simulink model "GAPID_NNPID_COMP"  (R2018a)
settings: Solver=FixedStepAuto  StartTime=0.0  StopTime=100  FixedStep=1e-3  RelTol=1e-3
model workspace (MAT data in the model file):
  Af = 3
  Cd = 0.38
  Cr = 0.01
  DrCycles.C505 = [0 1 2 3 4 5 6 7 8 9 10 11 ... (1012 elements, 506x2)]
  DrCycles.FTP = [0 1 2 3 4 5 6 7 8 9 10 11 ... (4956 elements, 2478x2)]
  DrCycles.UDDS = [0 1 2 3 4 5 6 7 8 9 10 11 ... (2746 elements, 1373x2)]
  DrCycles.HWFET = [0 1 2 3 4 5 6 7 8 9 10 11 ... (1532 elements, 766x2)]
  DrCycles.US06 = [0 1 2 3 4 5 6 7 8 9 10 11 ... (1194 elements, 597x2)]
  DrCycles.US06City = [0 1 2 3 4 5 6 7 8 9 10 11 ... (466 elements, 233x2)]
  DrCycles.US06Hwy = [0 1 2 3 4 5 6 7 8 9 10 11 ... (742 elements, 371x2)]
  I = 1
  Kbr = 5000
  M = 1500
  P = 20
  Sig = Simulink.Signal
  Sig.DataType = 'auto'
  Sig.Dimensions = -1
  Sig.DimensionsMode = 'auto'
  Sig.Complexity = 'auto'
  Sig.SampleTime = -1
  Sig.SamplingMode = 'auto'
  Sig1 = Simulink.Signal
  Sig1.DataType = 'auto'
  Sig1.Dimensions = -1
  Sig1.DimensionsMode = 'auto'
  Sig1.Complexity = 'auto'
  Sig1.SampleTime = -1
  Sig1.SamplingMode = 'auto'
  TimeHWFET = 765
  TimeUDDS = 1372
  TimeUS06 = 596
  W_h_o = [-9.95144559352  0.700876377684  31237.1112906; -121.542629392  0.870455912648  31044.7209619; -122.360742678  0.0476540509418  31044.6526126; -122.423418817  0.59044997874  31044.0707224]
  W_i_h = [0.80068585569  0.0488168547579  0.252518618973  0.0925761755134; 0.988834029296  0.225213340605  0.654342062876  0.334021271958; 0.439228284919  0.581023041467  0.0600961897607  0.651090707805; -0.495532270503  0.596404398277  0.940082136994  0.486403351376]
  axle_b = 10
  axle_k = 5000
  bevAxle_wc = 400
  bevNp = 2
  bevNs = 30
  diffRatio = 3.4
  g = 9.81
  m = 1500
  motorMaxTorqueNm = [500 500 500 500 500 500 416.666666667 357.142857143 312.5 277.777777778 250 227.272727273 208.333333333 192.307692308 178.571428571 166.666666667]
  motorSpeedRadPs = [0 40 80 120 160 200 240 280 320 360 400 440 480 520 560 600]
  rho = 1.28
  theta = 45
  vehicleMass = 1500
  wheelRadius = 0.35
values from neighbouring files (symbols this model uses):
  Kd = reshape(Kd,D1,D2,D3)    [Launch_Comparison.m]
  Ki = reshape(Ki,D1,D2,D3)    [Launch_Comparison.m]
  Kp = reshape(Kp,D1,D2,D3)    [Launch_Comparison.m]
  lr = 0.8    [Launch_Comparison.m]
  Theta = data(:,4)    [Launch_Comparison.m]
  Vref = data(:,6)    [Launch_Comparison.m]
  Vwind = data(:,5)    [Launch_Comparison.m]
undefined symbols (not defined in the file or in its folder): sigbuilder_block
libraries: simulink x4, autolibdatasheetbattery x2, autolibmappedmotor x2, autolibsharedcoupling x2, autolibshareddiff x2, autolibshared x2, Wheels_Driver_VehDyn_Lib x2
settings Model: OrderedModelArguments=off  Creator=Yacine.Kebbati  LastModifiedBy=yassi
settings DataIOCC: ReturnWorkspaceOutputs=on
settings SFSimCC: SimUseLocalCustomCode=on
settings RTWCC: RTWUseLocalCustomCode=on

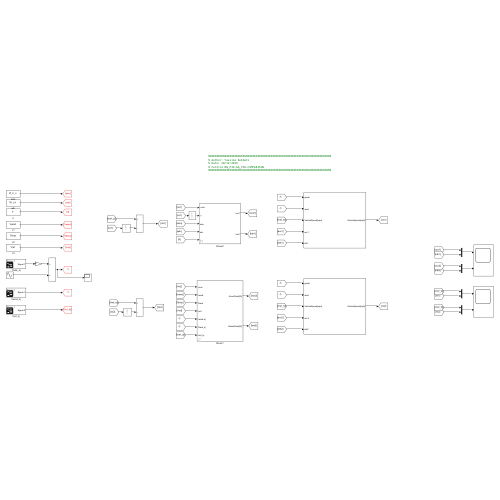
[thumbnail: Simulink's stored preview of the top-level diagram]
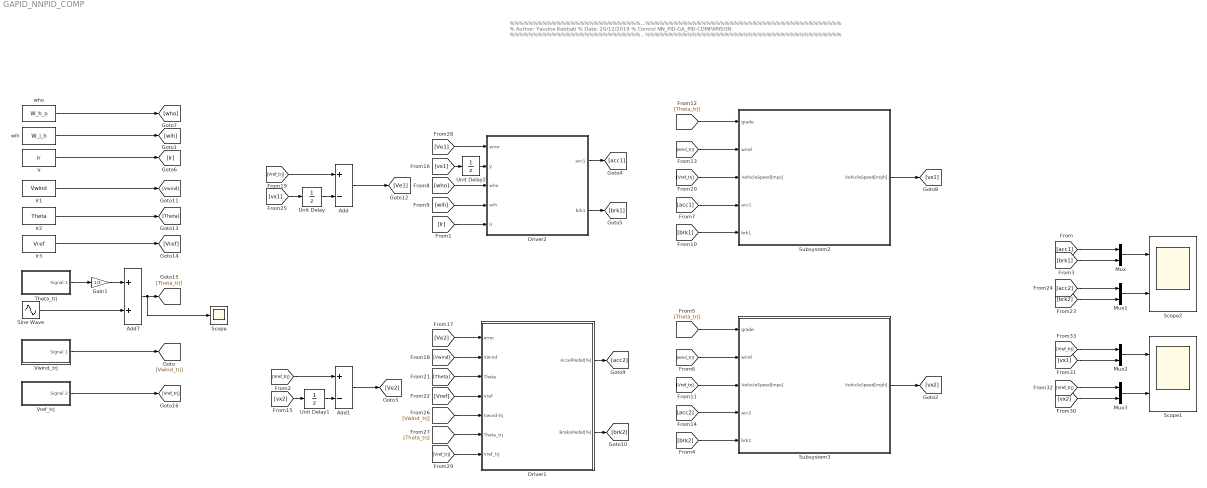
== system GAPID_NNPID_COMP ==
  note: %%%%%%%%%%%%%%%%%%%%%%%%%%%%%%%%%%%%%%%%%%%%%%%%%%%%%%%%%%%%%%%%%%%%%%%%%%%
      | % Author: Yassine Kebbati
      | % Date: 20/12/2019
      | % Control NN_PID-GA_PID-COMPARISON
      | %%%%%%%%%%%%%%%%%%%%%%%%%%%%%%%%%%%%%%%%%%%%%%%%%%%%%%%%%%%%%%%%%%%%%%%%%%%
  Add : Sum  Inputs=+-
  Add1 : Sum  Inputs=+-
  Add7 : Sum
  Driver1 : Subsystem  AncestorBlock=Wheels_Driver_VehDyn_Lib/Driver
  Driver2 : Subsystem  AncestorBlock=Wheels_Driver_VehDyn_Lib/Driver
  Gain1 : Gain  Gain=1/3
  Mux{,1..3} (4 alike) : Mux  Inputs=2
  Scope : Scope
  Scope1 : Scope  NumInputPorts=2
  Scope2 : Scope  NumInputPorts=2
  Sine Wave : Sin  Amplitude=4  Frequency=0.2  SampleTime=0
  Subsystem2 : Subsystem
  Subsystem3 : Subsystem
  Theta_trj : Subsystem  Tag=STV Subsys  LoadFcn=sigbuilder_block('load');  StartFcn=sigbuilder_block('start');  StopFcn=sigbuilder_block('stop');  ClipboardFcn=sigbuilder_block('clipboard');  mask(Sigbuilder block){tuvar=[0:10]}
      mask help: Simulink:masks:SigbuilderBlock_MD
      mask init:
      | if ~strcmp(get_param(bdroot(gcbh),'SimulationStatus'),'stopped') tuvar = sigbuilder_block('maskInit'); end
      settings: CopyFcn=sigbuilder_block('copy');  DeleteFcn=sigbuilder_block('delete');  ModelCloseFcn=sigbuilder_block('modelClose');  PreSaveFcn=sigbuilder_block('preSave');  PauseFcn=sigbuilder_block('pause');  ContinueFcn=sigbuilder_block('continue');  NameChangeFcn=sigbuilder_block('namechange');  OpenFcn=sigbuilder_block('open',[6 30 1428 681.75 ]);  CloseFcn=sigbuilder_block('close');
      mask Display: plot(0, 0, 100, 100,[2, 2, 32, 32, 2], [68, 8, 8, 68, 68],[32, 2], [38, 38], [32, 19, 2],[53, 60, 44], [32, 17, 17, 2],[16, 16, 31, 31]);txt = getActiveGroup(gcbh);text(2, 100, txt,'verticalAlignment', 'top');
  Unit Delay : UnitDelay  SampleTime=-1  HasFrameUpgradeWarning=on
  Unit Delay1 : UnitDelay  SampleTime=-1  HasFrameUpgradeWarning=on
  Unit Delay2 : UnitDelay  SampleTime=-1  HasFrameUpgradeWarning=on
  Vref_trj : Subsystem  Tag=STV Subsys  LoadFcn=sigbuilder_block('load');  StartFcn=sigbuilder_block('start');  StopFcn=sigbuilder_block('stop');  ClipboardFcn=sigbuilder_block('clipboard');  mask(Sigbuilder block){tuvar=[0:10]}
      mask help: Simulink:masks:SigbuilderBlock_MD
      mask init:
      | if ~strcmp(get_param(bdroot(gcbh),'SimulationStatus'),'stopped') tuvar = sigbuilder_block('maskInit'); end
      settings: CopyFcn=sigbuilder_block('copy');  DeleteFcn=sigbuilder_block('delete');  ModelCloseFcn=sigbuilder_block('modelClose');  PreSaveFcn=sigbuilder_block('preSave');  PauseFcn=sigbuilder_block('pause');  ContinueFcn=sigbuilder_block('continue');  NameChangeFcn=sigbuilder_block('namechange');  OpenFcn=sigbuilder_block('open',[0 36 1920 986.25 ]);  CloseFcn=sigbuilder_block('close');
      mask Display: plot(0, 0, 100, 100,[2, 2, 32, 32, 2], [68, 8, 8, 68, 68],[32, 2], [38, 38], [32, 19, 2],[53, 60, 44], [32, 17, 17, 2],[16, 16, 31, 31]);txt = getActiveGroup(gcbh);text(2, 100, txt,'verticalAlignment', 'top');
  Vwind_trj : Subsystem  Tag=STV Subsys  LoadFcn=sigbuilder_block('load');  StartFcn=sigbuilder_block('start');  StopFcn=sigbuilder_block('stop');  ClipboardFcn=sigbuilder_block('clipboard');  mask(Sigbuilder block){tuvar=[0:10]}
      mask help: Simulink:masks:SigbuilderBlock_MD
      mask init:
      | if ~strcmp(get_param(bdroot(gcbh),'SimulationStatus'),'stopped') tuvar = sigbuilder_block('maskInit'); end
      settings: CopyFcn=sigbuilder_block('copy');  DeleteFcn=sigbuilder_block('delete');  ModelCloseFcn=sigbuilder_block('modelClose');  PreSaveFcn=sigbuilder_block('preSave');  PauseFcn=sigbuilder_block('pause');  ContinueFcn=sigbuilder_block('continue');  NameChangeFcn=sigbuilder_block('namechange');  OpenFcn=sigbuilder_block('open',[140.25 245.25 1428 681.75 ]);  CloseFcn=sigbuilder_block('close');
      mask Display: plot(0, 0, 100, 100,[2, 2, 32, 32, 2], [68, 8, 8, 68, 68],[32, 2], [38, 38], [32, 19, 2],[53, 60, 44], [32, 17, 17, 2],[16, 16, 31, 31]);txt = getActiveGroup(gcbh);text(2, 100, txt,'verticalAlignment', 'top');
  lr : Constant  Value=lr  SampleTime=-1
  lr1 : Constant  Value=Vwind  SampleTime=-1
  lr2 : Constant  Value=Theta  SampleTime=-1
  lr3 : Constant  Value=Vref  SampleTime=-1
  who : Constant  Value=W_h_o  SampleTime=-1
  wih : Constant  Value=W_i_h  SampleTime=-1
  wires:
  [Theta_trj] -> Subsystem2/1(grade)
  Driver2/1(acc1) -> [acc1]
  [vx1] -> Unit Delay/1
  Add/1 -> [Ve1]
  [Vref_trj] -> Subsystem2/3(VehicleSpeed[mps])
  [Vref_trj] -> Add/1
  [acc1] -> Subsystem2/4(acc1)
  [brk1] -> Subsystem2/5(brk1)
  Subsystem2/1(VehicleSpeed[mph]) -> [vx1]
  Driver2/2(brk1) -> [brk1]
  [wind_trj] -> Subsystem2/2(wind)
  [vx1] -> Unit Delay2/1
  [Ve1] -> Driver2/1(" error")
  who/1 -> [who]
  wih/1 -> [wih]
  lr/1 -> [lr]
  [who] -> Driver2/3(who)
  [wih] -> Driver2/4(wih)
  [lr] -> Driver2/5(lr)
  Mux1/1 -> Scope2/2
  Mux/1 -> Scope2/1
  [acc1] -> Mux/1
  [brk1] -> Mux/2
  Subsystem3/1(VehicleSpeed[mph]) -> [vx2]
  [acc2] -> Subsystem3/4(acc2)
  [wind_trj] -> Subsystem3/2(wind)
  [brk2] -> Subsystem3/5(brk2)
  [Theta_trj] -> Subsystem3/1(grade)
  [Vref_trj] -> Subsystem3/3(VehicleSpeed[mps])
  [Vref_trj] -> Add1/1
  Add1/1 -> [Ve2]
  [vx2] -> Unit Delay1/1
  [Ve2] -> Driver1/1(" error")
  Driver1/1(AccelPedal[%]) -> [acc2]
  Driver1/2(BrakePedal[%]) -> [brk2]
  [Vwind] -> Driver1/2(Vwind)
  [Theta] -> Driver1/3(Theta)
  [Vref] -> Driver1/4(Vref)
  [acc2] -> Mux1/1
  [brk2] -> Mux1/2
  lr1/1 -> [Vwind]
  lr3/1 -> [Vref]
  lr2/1 -> [Theta]
  [Vwind_trj] -> Driver1/5(Vwind-trj)
  [Theta_trj] -> Driver1/6(Theta_trj)
  [Vref_trj] -> Driver1/7(Vref_trj)
  Sine Wave/1 -> Add7/2
  Gain1/1 -> Add7/1
  Theta_trj/1(Signal 1) -> Gain1/1
  Add7/1 -> Scope/1, [Theta_trj]
  Vwind_trj/1(Signal 1) -> [Vwind_trj]
  Vref_trj/1(Signal 2) -> [Vref_trj]
  Unit Delay/1 -> Add/2
  Unit Delay1/1 -> Add1/2
  Unit Delay2/1 -> Driver2/2(" y")
  [vx2] -> Mux3/2
  [Vref_trj] -> Mux3/1
  [vx1] -> Mux2/2
  [Vref_trj] -> Mux2/1
  Mux2/1 -> Scope1/1
  Mux3/1 -> Scope1/2

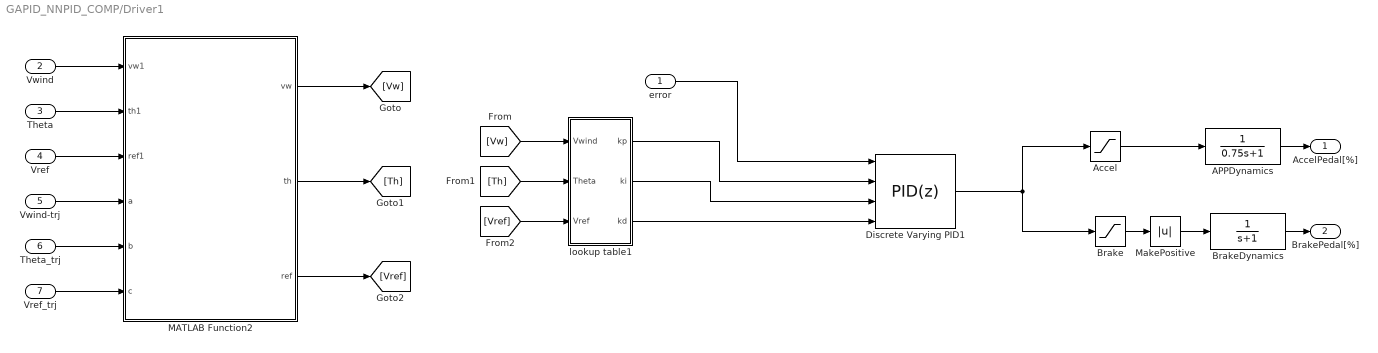
== system GAPID_NNPID_COMP/Driver1 ==
  " error" : Inport
  Vwind : Inport  Port=2
  Theta : Inport  Port=3
  Vref : Inport  Port=4
  Vwind-trj : Inport  Port=5
  Theta_trj : Inport  Port=6
  Vref_trj : Inport  Port=7
  APPDynamics : TransferFcn  Denominator=[0.75 1]
  Accel : Saturate  UpperLimit=100  LowerLimit=0
  Brake : Saturate  UpperLimit=0  LowerLimit=-100
  BrakeDynamics : TransferFcn  Denominator=[1 1]
  Discrete Varying PID1 : simulink/Continuous/PID Controller  Controller=PID  Form=Parallel  TimeDomain=Discrete-time  SampleTime=-1  IntegratorMethod=Forward Euler  ControllerParametersSource=external  P=1  I=1  D=0  N=100  UseFilter=off  TunerSelectOption=Transfer Function Based (PID Tuner App)  InitialConditionSource=internal  InitialConditionForIntegrator=0  InitialConditionForFilter=0  DifferentiatorICPrevScaledInput=0  ExternalReset=none  TrackingMode=off  Kt=1  LimitOutput=off  UpperSaturationLimit=100  LowerSaturationLimit=-100  LinearizeAsGain=on  AntiWindupMode=none  Kb=1  POutMin=[]  POutMax=[]  IOutMin=[]  IOutMax=[]  DOutMin=[]  DOutMax=[]  NOutMin=[]  NOutMax=[]  SumOutMin=[]  SumOutMax=[]  SaturationOutMin=[]  SaturationOutMax=[]  PParamMin=[]  PParamMax=[]  IParamMin=[]  IParamMax=[]  DParamMin=[]  DParamMax=[]  NParamMin=[]  NParamMax=[]  KbParamMin=[]  KbParamMax=[]  KtParamMin=[]  KtParamMax=[]  KbOutMin=[]  KbOutMax=[]  KtOutMin=[]  KtOutMax=[]  IntegratorOutMin=[]  IntegratorOutMax=[]  FilterOutMin=[]  FilterOutMax=[]  SumI1OutMin=[]  SumI1OutMax=[]  SumI2OutMin=[]  SumI2OutMax=[]  SumI3OutMin=[]  SumI3OutMax=[]  SumDOutMin=[]  SumDOutMax=[]  DifferentiatorOutMin=[]  DifferentiatorOutMax=[]  FilterDiffOutCoefMin=[]  FilterDiffOutCoefMax=[]  ReciprocalOutMin=[]  ReciprocalOutMax=[]  SumDenOutMin=[]  SumDenOutMax=[]  SumNumOutMin=[]  SumNumOutMax=[]  DivideOutMin=[]  DivideOutMax=[]  IntegratorContinuousStateAttributes=''  IntegratorStateMustResolveToSignalObject=off  IntegratorRTWStateStorageClass=Auto  FilterContinuousStateAttributes=''  FilterStateMustResolveToSignalObject=off  FilterRTWStateStorageClass=Auto
  MATLAB Function2 : MATLAB Function  TreatAsAtomicUnit=on
  MakePositive : Abs
  lookup table1 : Subsystem
  AccelPedal[%] : Outport  VectorParamsAs1DForOutWhenUnconnected=off
  BrakePedal[%] : Outport  Port=2  VectorParamsAs1DForOutWhenUnconnected=off
  wires:
  Discrete Varying PID1/1 -> Brake/1, Accel/1
  APPDynamics/1 -> AccelPedal[%]/1
  BrakeDynamics/1 -> BrakePedal[%]/1
  Brake/1 -> MakePositive/1
  Accel/1 -> APPDynamics/1
  MakePositive/1 -> BrakeDynamics/1
  lookup table1/2(ki) -> Discrete Varying PID1/3
  lookup table1/3("kd ") -> Discrete Varying PID1/4
  lookup table1/1(kp) -> Discrete Varying PID1/2
  " error"/1 -> Discrete Varying PID1/1
  [Vw] -> lookup table1/1(Vwind)
  [Th] -> lookup table1/2(Theta)
  [Vref] -> lookup table1/3(Vref)
  Vwind/1 -> MATLAB Function2/1(vw1)
  Theta/1 -> MATLAB Function2/2(th1)
  Vref/1 -> MATLAB Function2/3(ref1)
  MATLAB Function2/1(vw) -> [Vw]
  MATLAB Function2/2(th) -> [Th]
  MATLAB Function2/3(ref) -> [Vref]
  Vref_trj/1 -> MATLAB Function2/6(c)
  Theta_trj/1 -> MATLAB Function2/5(b)
  Vwind-trj/1 -> MATLAB Function2/4(a)

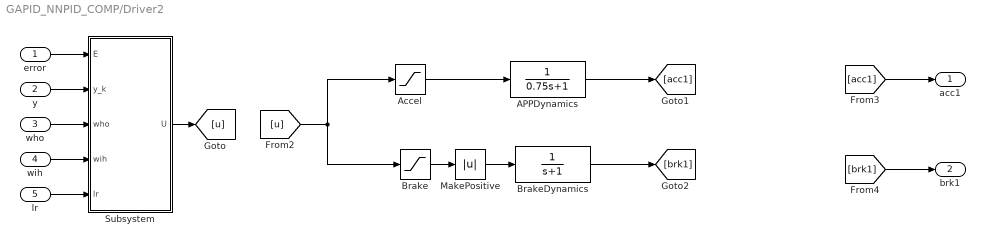
== system GAPID_NNPID_COMP/Driver2 ==
  " error" : Inport
  " y" : Inport  Port=2
  who : Inport  Port=3
  wih : Inport  Port=4
  lr : Inport  Port=5
  APPDynamics : TransferFcn  Denominator=[0.75 1]
  Accel : Saturate  UpperLimit=100  LowerLimit=0
  Brake : Saturate  UpperLimit=0  LowerLimit=-100
  BrakeDynamics : TransferFcn  Denominator=[1 1]
  MakePositive : Abs
  Subsystem : Subsystem
  acc1 : Outport  VectorParamsAs1DForOutWhenUnconnected=off
  brk1 : Outport  Port=2  VectorParamsAs1DForOutWhenUnconnected=off
  wires:
  MakePositive/1 -> BrakeDynamics/1
  " error"/1 -> Subsystem/1(E)
  Accel/1 -> APPDynamics/1
  Brake/1 -> MakePositive/1
  " y"/1 -> Subsystem/2(y_k)
  BrakeDynamics/1 -> [brk1]
  APPDynamics/1 -> [acc1]
  [u] -> Accel/1, Brake/1
  Subsystem/1(U) -> [u]
  [acc1] -> acc1/1
  [brk1] -> brk1/1
  who/1 -> Subsystem/3(who)
  wih/1 -> Subsystem/4(wih)
  lr/1 -> Subsystem/5(lr)

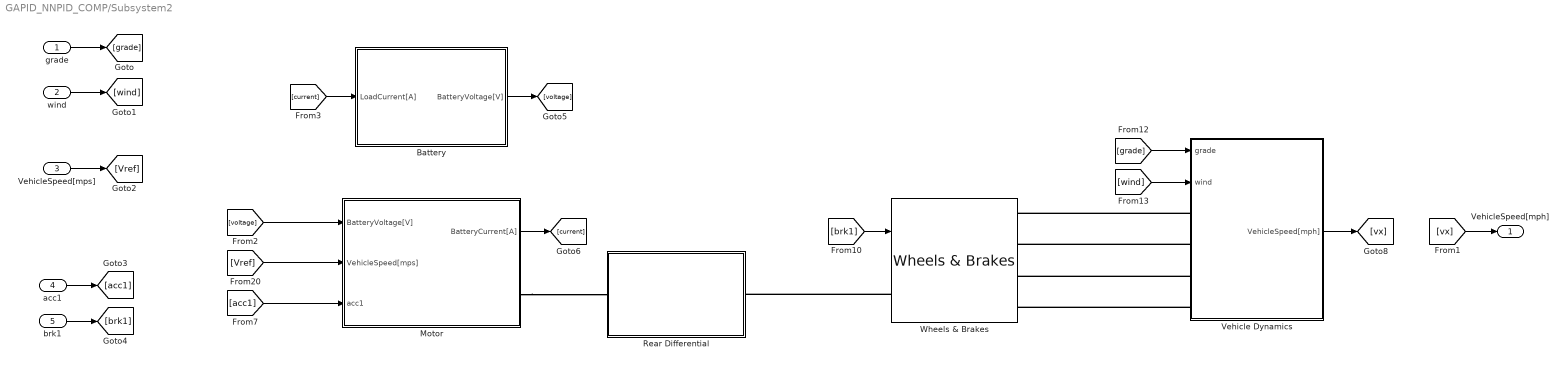
== system GAPID_NNPID_COMP/Subsystem2 ==
  grade : Inport
  wind : Inport  Port=2
  VehicleSpeed[mps] : Inport  Port=3
  acc1 : Inport  Port=4
  brk1 : Inport  Port=5
  Battery : Subsystem
  Motor : Subsystem
  Rear Differential : Subsystem
  Vehicle Dynamics : Subsystem  AncestorBlock=Wheels_Driver_VehDyn_Lib/Vehicle Dynamics
  "Wheels & Brakes " : Wheels_Driver_VehDyn_Lib/Wheels & Brakes  SystemSampleTime=-1  Latency=0  AutoFrameSizeCalculation=off
      link override BrakeGain: Gain=Kbr
      link override Longitudinal Wheel - Disk Brake: Re=0.32995  Lrel=0.32995  rollingType=Magic Formula  Iyy=0.798  UNLOADED_RADIUS=0.32995  num_pads=2
      link override Longitudinal Wheel - Disk Brake1: Iyy=0.798  Lrel=0.32995  Re=0.32995  rollingType=Magic Formula  UNLOADED_RADIUS=0.32995
  VehicleSpeed[mph] : Outport
  wires:
  [wind] -> Vehicle Dynamics/2(wind)
  [current] -> Battery/1(LoadCurrent[A])
  [voltage] -> Motor/1(BatteryVoltage[V])
  [grade] -> Vehicle Dynamics/1(grade)
  [vx] -> VehicleSpeed[mph]/1
  [brk1] -> "Wheels & Brakes "/1
  [Vref] -> Motor/2(VehicleSpeed[mps])
  [acc1] -> Motor/3(acc1)
  Vehicle Dynamics/1(VehicleSpeed[mph]) -> [vx]
  grade/1 -> [grade]
  wind/1 -> [wind]
  VehicleSpeed[mps]/1 -> [Vref]
  acc1/1 -> [acc1]
  brk1/1 -> [brk1]
  Battery/1(BatteryVoltage[V]) -> [voltage]
  Motor/1(BatteryCurrent[A]) -> [current]
  connections:
  Motor/RConn1 -- Rear Differential/LConn1
  Vehicle Dynamics/LConn4 -- "Wheels & Brakes "/RConn4
  Vehicle Dynamics/LConn2 -- "Wheels & Brakes "/RConn2
  Vehicle Dynamics/LConn1 -- "Wheels & Brakes "/RConn1
  Vehicle Dynamics/LConn3 -- "Wheels & Brakes "/RConn3
  "Wheels & Brakes "/LConn1 -- Rear Differential/RConn1

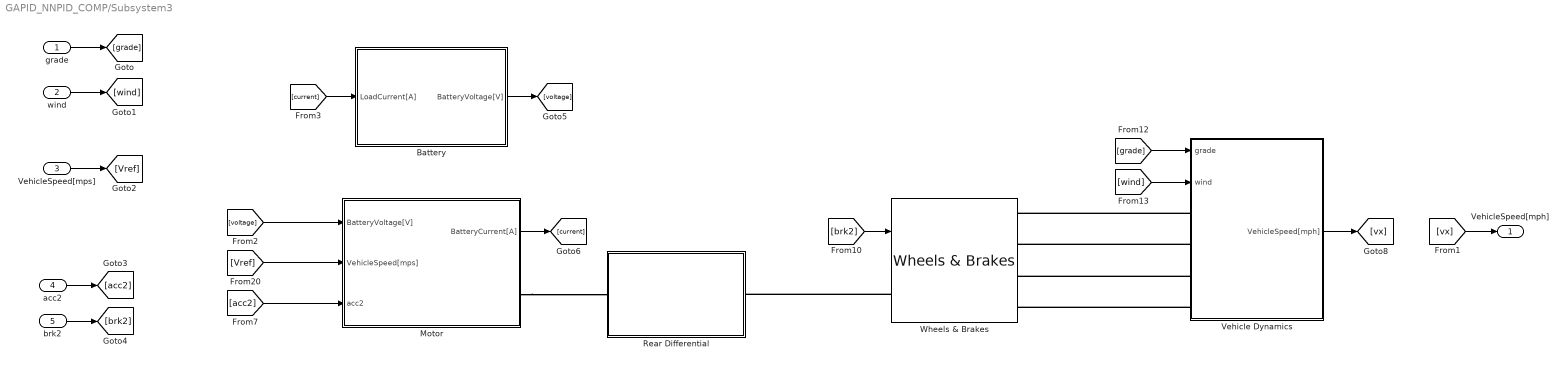
== system GAPID_NNPID_COMP/Subsystem3 ==
  grade : Inport
  wind : Inport  Port=2
  VehicleSpeed[mps] : Inport  Port=3
  acc2 : Inport  Port=4
  brk2 : Inport  Port=5
  Battery : Subsystem
  Motor : Subsystem
  Rear Differential : Subsystem
  Vehicle Dynamics : Subsystem  AncestorBlock=Wheels_Driver_VehDyn_Lib/Vehicle Dynamics
  "Wheels & Brakes " : Wheels_Driver_VehDyn_Lib/Wheels & Brakes  SystemSampleTime=-1  Latency=0  AutoFrameSizeCalculation=off
      link override BrakeGain: Gain=Kbr
      link override Longitudinal Wheel - Disk Brake: Re=0.32995  Lrel=0.32995  rollingType=Magic Formula  Iyy=0.798  UNLOADED_RADIUS=0.32995  num_pads=2
      link override Longitudinal Wheel - Disk Brake1: Iyy=0.798  Lrel=0.32995  Re=0.32995  rollingType=Magic Formula  UNLOADED_RADIUS=0.32995
  VehicleSpeed[mph] : Outport
  wires:
  [wind] -> Vehicle Dynamics/2(wind)
  [current] -> Battery/1(LoadCurrent[A])
  [voltage] -> Motor/1(BatteryVoltage[V])
  [grade] -> Vehicle Dynamics/1(grade)
  [vx] -> VehicleSpeed[mph]/1
  [brk2] -> "Wheels & Brakes "/1
  [Vref] -> Motor/2(VehicleSpeed[mps])
  [acc2] -> Motor/3(acc2)
  Vehicle Dynamics/1(VehicleSpeed[mph]) -> [vx]
  grade/1 -> [grade]
  wind/1 -> [wind]
  VehicleSpeed[mps]/1 -> [Vref]
  acc2/1 -> [acc2]
  brk2/1 -> [brk2]
  Battery/1(BatteryVoltage[V]) -> [voltage]
  Motor/1(BatteryCurrent[A]) -> [current]
  connections:
  Motor/RConn1 -- Rear Differential/LConn1
  Vehicle Dynamics/LConn4 -- "Wheels & Brakes "/RConn4
  Vehicle Dynamics/LConn2 -- "Wheels & Brakes "/RConn2
  Vehicle Dynamics/LConn1 -- "Wheels & Brakes "/RConn1
  Vehicle Dynamics/LConn3 -- "Wheels & Brakes "/RConn3
  "Wheels & Brakes "/LConn1 -- Rear Differential/RConn1

== system GAPID_NNPID_COMP/Theta_trj ==
  Demux : Demux  Tag=STV Demux  Outputs=1
      settings: DisplayOption=none
  FromWs : FromWorkspace  Tag=STV FromWs  VariableName=tuvar
      SigBuilderData=|
      | common.afterFinalStr = 'Extrapolate'
      | common.sampleTime = 0
      | dataSet.timeRange = [0 100]
      | dataSet.name = 'Group 1'
      | sbobj.Groups.Name = 'Group 1'
      | sbobj.Groups.Signals.Name = 'Signal 1'
      | sbobj.Groups.Signals.XData = [0 1.2 2.2 3.2 4.2 5.2 6.2 7.2 8.2 9.2 10.2 11.2 12.2 13.2 14.2 15.2 16.2 17.2 18.2 19.2 20.2 21.2 22.2 23.2 24.2 25.2 26.2 27.2 28.2 29.2 30.2 31.2 32.2 33.2 34.2 35.2 36.2 37.2 38.2 39.2 40.2 41.2 42.2 43.2 44.2 45.2 46.2 47.2 48.2 49.2 50.2 51.2 52.2 53.2 54.2 55.2 56.2 57.2 58.2 59.2 60.2 61.2 62.2 63.2 64.2 65.2 66.2 67.2 68.2 69.2 70.2 71.2 72.2 73.2 74.2 75.2 76.2 77.2 78.2 79.2 80.2 81.2 82.2 83.2 84.2 85.2 86.2 87.2 88.2 89.2 90.2 91.2 92.2 93.2 94.2 95.2 96.2 97.2 98.2 100]
      | sbobj.Groups.Signals.YData = [9.95 9.95 9.95 9.95 9.95 9.95 9.95 10 10.1 10.15 10.45 10.95 11.95 12.95 13.95 14.95 15.95 16.95 17.95 18.95 19.95 20.95 21.95 22.95 23.95 24.45 24.75 24.95 24.95 24.95 24.95 24.95 24.95 24.95 24.9 24.65 24.4 24.05 23.1 21.8 20.95 19.9 18.65 18.1 17.3 15.95 14.55 13.5 12.2 11.3 10.7 10.1 9.95 9.95 9.95 9.95 9.95 9.95 9.95 9.95 9.8 9.55 8.8 7.95 6.95 5.95 4.95 3.95 3.3 2.5 2.05 1.95 1.95 1.95 1.95 1.95 1.95 1.95 1.95 1.95 2.15 2.4 2.5 2.8 3.1 3.45 3.95 4.45 4.7 4.75 4.75 4.8 4.95 4.95 4.95 4.95 4.95 4.95 4.95 4.95]
      | sbobj.Groups.TimeRange = [0 100]
  Signal 1 : Outport  Tag=STV Outport
  wires:
  Demux/1 -> Signal 1/1
  FromWs/1 -> Demux/1

== system GAPID_NNPID_COMP/Vref_trj ==
  Demux : Demux  Tag=STV Demux  Outputs=1
      settings: DisplayOption=none
  FromWs : FromWorkspace  Tag=STV FromWs  VariableName=tuvar
      SigBuilderData=|
      | common.afterFinalStr = 'Extrapolate'
      | common.sampleTime = 0
      | dataSet.timeRange = [0 99]
      | dataSet.name = 'Group 1'
      | sbobj.Groups.Name = 'Group 1'
      | sbobj.Groups.Signals.Name = 'Signal 2'
      | sbobj.Groups.Signals.XData = [0 1.2 2.2 3.2 4.2 5.2 6.2 7.2 8.2 9.2 10.2 11.2 12.2 13.2 14.2 15.2 16.2 17.2 18.2 19.2 20.2 21.2 22.2 23.2 24.2 25.2 26.2 27.2 28.2 29.2 30.2 31.2 32.2 33.2 34.2 35.2 36.2 37.2 38.2 39.2 40.2 41.2 42.4 43.2 44.2 45.2 46.2 47.2 48.2 49.2 50.2 51.2 52.2 53.2 54.2 55.2 56.2 57.2 58.2 59.2 60.2 61.2 62.2 63.2 64.2 65.2 66.2 67.2 68.2 69.2 70.2 71.2 72.2 73.2 74.2 75.2 76.2 77.2 78.2 79.2 80.2 81.2 82.2 83.2 84.2 85.2 86.2 87.2 88.2 89.2 90.2 91.2 92.2 93.2 94.2 95.2 96.2 97.2 98.2 99]
      | sbobj.Groups.Signals.YData = [2 2.35 2.75 3.5 4.25 4.8 5.75 6 6.05 4.35 3.7 3.55 3.65 4.2 4.9 5.05 4.65 4.9 6.4 7.95 10.45 12 12.5 12.75 12.4 12 11.55 10.95 11 11.05 11.55 12 12 12.3 12.55 13.3 13.7 13.6 13.9 14.9 15.85 16.95 17.6 17.7 18.3 18.65 18.95 19.5 19.7 20.4 21.65 22.35 22.8 22.7 22.75 22.35 22.45 23.2 23.45 23.6 23.8 23.75 23.95 24.55 25.1 25.1 25.4 25.65 25.9 25.75 25.3 25.15 24.55 23.85 23.25 22.6 22.2 21.6 20.85 19.85 18 16 14.45 13.85 13.25 12.9 12.4 12.1 11.85 11.45 10.7 10.55 9.95 9.75 9.75 9.75 9.75 9.75 9.75 9.75]
      | sbobj.Groups.TimeRange = [0 99]
  Signal 2 : Outport  Tag=STV Outport
  wires:
  FromWs/1 -> Demux/1
  Demux/1 -> Signal 2/1

== system GAPID_NNPID_COMP/Vwind_trj ==
  Demux : Demux  Tag=STV Demux  Outputs=1
      settings: DisplayOption=none
  FromWs : FromWorkspace  Tag=STV FromWs  VariableName=tuvar
      SigBuilderData=|
      | common.afterFinalStr = 'Extrapolate'
      | common.sampleTime = 0
      | dataSet.timeRange = [0 100]
      | dataSet.name = 'Group 1'
      | sbobj.Groups.Name = 'Group 1'
      | sbobj.Groups.Signals.Name = 'Signal 1'
      | sbobj.Groups.Signals.XData = [0 1.2 2.2 3.2 4.2 5.2 6.2 7.2 8.2 9.2 10.2 11.2 12.2 13.2 14.2 15.2 16.2 17.2 18.2 19.2 20.2 21.2 22.2 23.2 24.2 25.2 26.2 27.2 28.2 29.2 30.2 31.2 32.2 33.2 34.2 35.2 36.2 37.2 38.2 39.2 40.2 41.2 42.2 43.2 44.2 45.2 46.2 47.2 48.2 49.2 50.2 51.2 52.2 53.2 54.2 55.2 56.2 57.2 58.2 59.2 60.2 61.2 62.2 63.2 64.2 65.2 66.2 67.2 68.2 69.2 70.2 71.2 72.2 73.2 74.2 75.2 76.2 77.2 78.2 79.2 80.2 81.2 82.2 83.2 84.2 85.2 86.2 87.2 88.2 89.2 90.2 91.2 92.2 93.2 94.2 95.2 96.2 97.2 98.2 100]
      | sbobj.Groups.Signals.YData = [2.35 2.35 2.35 2.35 2.35 2.35 2.35 2.35 2.35 2.35 2.35 2.35 2.35 2.35 2.35 2.35 2.35 2.35 2.35 2.35 8.35 8.35 8.35 8.35 8.35 8.35 8.35 8.35 8.35 8.35 8.35 8.35 8.35 8.35 8.35 8.35 8.35 8.35 8.35 8.35 20.35 20.35 20.35 20.35 20.35 20.35 20.35 20.35 20.35 20.35 20.35 20.35 20.35 20.35 20.35 20.35 20.35 20.35 20.35 20.35 25.35 25.35 25.35 25.35 25.35 25.35 25.35 25.35 25.35 25.35 25.35 25.35 25.35 25.35 25.35 25.35 25.35 25.35 25.35 25.35 15.35 15.35 15.35 15.35 15.35 15.35 15.35 15.35 15.35 15.35 15.35 15.35 15.35 15.35 15.35 15.35 15.35 15.35 15.35 15.35]
      | sbobj.Groups.TimeRange = [0 100]
  Signal 1 : Outport  Tag=STV Outport
  wires:
  FromWs/1 -> Demux/1
  Demux/1 -> Signal 1/1

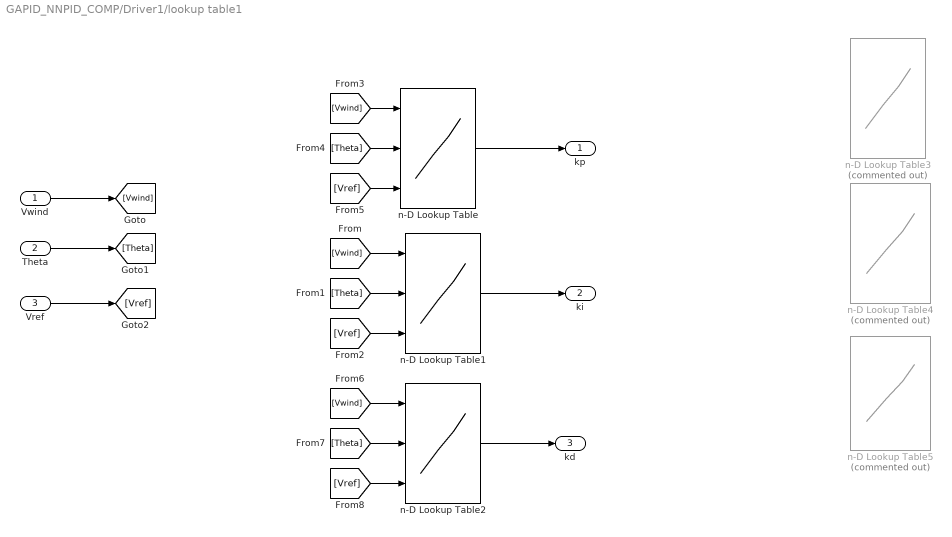
== system GAPID_NNPID_COMP/Driver1/lookup table1 ==
  Vwind : Inport
  Theta : Inport  Port=2
  Vref : Inport  Port=3
  n-D Lookup Table : Lookup_n-D  NumberOfTableDimensions=3  BreakpointsForDimension1=0:1.15:20  BreakpointsForDimension2=0:1.2:20  BreakpointsForDimension3=5:1.4:30  Table=Kp  InternalRulePriority=Speed  RndMeth=Simplest  InputSameDT=on
  n-D Lookup Table1 : Lookup_n-D  NumberOfTableDimensions=3  BreakpointsForDimension1=0:1.15:20  BreakpointsForDimension2=0:1.2:20  BreakpointsForDimension3=5:1.4:30  Table=Ki  InternalRulePriority=Speed  RndMeth=Simplest  InputSameDT=on
  n-D Lookup Table2 : Lookup_n-D  NumberOfTableDimensions=3  BreakpointsForDimension1=0:1.15:20  BreakpointsForDimension2=0:1.2:20  BreakpointsForDimension3=5:1.4:30  Table=Kd  InternalRulePriority=Speed  RndMeth=Simplest  InputSameDT=on
  n-D Lookup Table3 : Lookup_n-D  Commented=on  NumberOfTableDimensions=3  BreakpointsForDimension1=-15:2.5:15  BreakpointsForDimension2=-20:2.6:20  BreakpointsForDimension3=0:1.8:30  Table=Kp  InternalRulePriority=Speed  RndMeth=Simplest  InputSameDT=on
  n-D Lookup Table4 : Lookup_n-D  Commented=on  NumberOfTableDimensions=3  BreakpointsForDimension1=-15:2.5:15  BreakpointsForDimension2=-20:2.6:20  BreakpointsForDimension3=0:1.8:30  Table=Ki  InternalRulePriority=Speed  RndMeth=Simplest  InputSameDT=on
  n-D Lookup Table5 : Lookup_n-D  Commented=on  NumberOfTableDimensions=3  BreakpointsForDimension1=-15:2.5:15  BreakpointsForDimension2=-20:2.6:20  BreakpointsForDimension3=0:1.8:30  Table=Kd  InternalRulePriority=Speed  RndMeth=Simplest  InputSameDT=on
  kp : Outport
  ki : Outport  Port=2
  "kd " : Outport  Port=3
  wires:
  n-D Lookup Table/1 -> kp/1
  n-D Lookup Table1/1 -> ki/1
  n-D Lookup Table2/1 -> "kd "/1
  Vwind/1 -> [Vwind]
  Theta/1 -> [Theta]
  Vref/1 -> [Vref]
  [Vref] -> n-D Lookup Table1/3
  [Theta] -> n-D Lookup Table1/2
  [Vwind] -> n-D Lookup Table1/1
  [Vref] -> n-D Lookup Table/3
  [Theta] -> n-D Lookup Table/2
  [Vwind] -> n-D Lookup Table/1
  [Vref] -> n-D Lookup Table2/3
  [Theta] -> n-D Lookup Table2/2
  [Vwind] -> n-D Lookup Table2/1

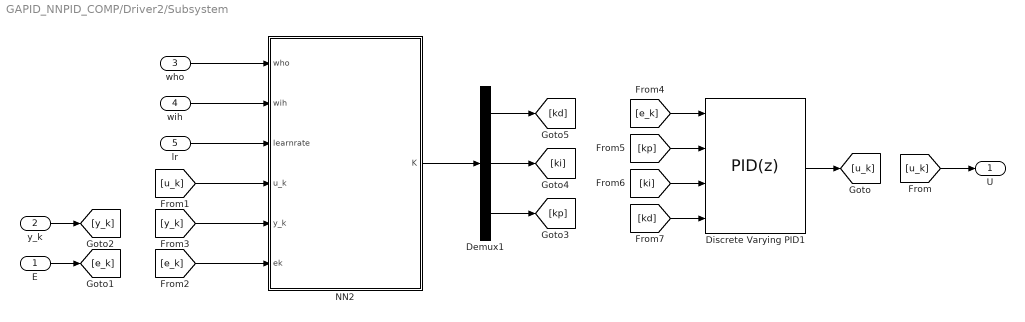
== system GAPID_NNPID_COMP/Driver2/Subsystem ==
  E : Inport
  y_k : Inport  Port=2
  who : Inport  Port=3
  wih : Inport  Port=4
  lr : Inport  Port=5
  Demux1 : Demux  Outputs=3
  Discrete Varying PID1 : simulink/Continuous/PID Controller  Controller=PID  Form=Parallel  TimeDomain=Discrete-time  SampleTime=-1  IntegratorMethod=Forward Euler  ControllerParametersSource=external  P=1  I=1  D=0  N=100  UseFilter=off  TunerSelectOption=Transfer Function Based (PID Tuner App)  InitialConditionSource=internal  InitialConditionForIntegrator=0  InitialConditionForFilter=0  DifferentiatorICPrevScaledInput=0  ExternalReset=none  TrackingMode=off  Kt=1  LimitOutput=off  UpperSaturationLimit=100  LowerSaturationLimit=-100  LinearizeAsGain=on  AntiWindupMode=none  Kb=1  POutMin=[]  POutMax=[]  IOutMin=[]  IOutMax=[]  DOutMin=[]  DOutMax=[]  NOutMin=[]  NOutMax=[]  SumOutMin=[]  SumOutMax=[]  SaturationOutMin=[]  SaturationOutMax=[]  PParamMin=[]  PParamMax=[]  IParamMin=[]  IParamMax=[]  DParamMin=[]  DParamMax=[]  NParamMin=[]  NParamMax=[]  KbParamMin=[]  KbParamMax=[]  KtParamMin=[]  KtParamMax=[]  KbOutMin=[]  KbOutMax=[]  KtOutMin=[]  KtOutMax=[]  IntegratorOutMin=[]  IntegratorOutMax=[]  FilterOutMin=[]  FilterOutMax=[]  SumI1OutMin=[]  SumI1OutMax=[]  SumI2OutMin=[]  SumI2OutMax=[]  SumI3OutMin=[]  SumI3OutMax=[]  SumDOutMin=[]  SumDOutMax=[]  DifferentiatorOutMin=[]  DifferentiatorOutMax=[]  FilterDiffOutCoefMin=[]  FilterDiffOutCoefMax=[]  ReciprocalOutMin=[]  ReciprocalOutMax=[]  SumDenOutMin=[]  SumDenOutMax=[]  SumNumOutMin=[]  SumNumOutMax=[]  DivideOutMin=[]  DivideOutMax=[]  IntegratorContinuousStateAttributes=''  IntegratorStateMustResolveToSignalObject=off  IntegratorRTWStateStorageClass=Auto  FilterContinuousStateAttributes=''  FilterStateMustResolveToSignalObject=off  FilterRTWStateStorageClass=Auto
  NN2 : Subsystem
  U : Outport
  wires:
  lr/1 -> NN2/3(learnrate)
  who/1 -> NN2/1(who)
  [u_k] -> U/1
  wih/1 -> NN2/2(wih)
  [e_k] -> NN2/6(ek)
  NN2/1(K) -> Demux1/1
  [y_k] -> NN2/5(y_k)
  Discrete Varying PID1/1 -> [u_k]
  [u_k] -> NN2/4(u_k)
  [e_k] -> Discrete Varying PID1/1
  Demux1/3 -> [kp]
  Demux1/2 -> [ki]
  Demux1/1 -> [kd]
  [kp] -> Discrete Varying PID1/2
  [ki] -> Discrete Varying PID1/3
  [kd] -> Discrete Varying PID1/4
  y_k/1 -> [y_k]
  E/1 -> [e_k]

== system GAPID_NNPID_COMP/Subsystem2/Battery ==
  LoadCurrent[A] : Inport
  AmbientTemp[C] : Constant  Value=27
  Bus Selector : BusSelector  OutputSignals=BattSoc
  C2K : Bias  Bias=273
  Datasheet Battery : autolibdatasheetbattery/Datasheet Battery  CapacityCtrl=Parameter  OutputVlt=Unfiltered  BattChargeMax=131.82  Em=[3.167 3.413 3.446 3.488 3.537 3.571 3.593 3.610 3.625 3.642 3.663 3.695 3.755 3.799 3.846 3.895 3.945 3.997 4.051 4.108 4.166]  CapLUTBp=[0 0.05 0.1 0.15 0.2 0.25 0.3 0.35 0.4 0.45 0.5 0.55 0.6 0.65 0.7 0.75 0.8 0.85 0.9 0.95 1]  RInt=[0.008846 0.009319 0.009027 0.00847 0.01032 0.01314;0.006389 0.006554 0.005553 0.005525 0.006043 0.007805;0.004364 0.004101 0.00406 0.003452 0.003846 0.004517;0.002031 0.002563 0.002532 0.00246 0.002716 0.003047;0.001443 0.001825 0.001795 0.001778 0.001924 0.002234;0.0005603 0.0007192 0.0006887 0.0007557 0.0007355 0.001014;0.001028 0.001338 0.001 0.001536 0.001546 0.002789]  BattTempBp=[243.1 253.1 263.1 273.1 283.1 298.1 313.1]  CapSOCBp=[0 0.2 0.4 0.6 0.8 1]  Ns=96  Np=2  BattCapInit=131.82  Tc=1/1000  Vinit=4.221
  SOCto% : Gain  Gain=100
  Scope : Scope
  Stop Simulation : Stop
  lowSOClimit : simulink/Logic and Bit Operations/Compare To Constant  relop=<=  const=5  OutDataTypeStr=boolean
  BatteryVoltage[V] : Outport  VectorParamsAs1DForOutWhenUnconnected=off
  wires:
  Datasheet Battery/1 -> Bus Selector/1
  AmbientTemp[C]/1 -> C2K/1
  Datasheet Battery/2 -> BatteryVoltage[V]/1
  C2K/1 -> Datasheet Battery/2
  SOCto%/1 -> lowSOClimit/1, Scope/1
  Bus Selector/1 -> SOCto%/1  "<BattSoc>"
  LoadCurrent[A]/1 -> Datasheet Battery/1
  lowSOClimit/1 -> Stop Simulation/1

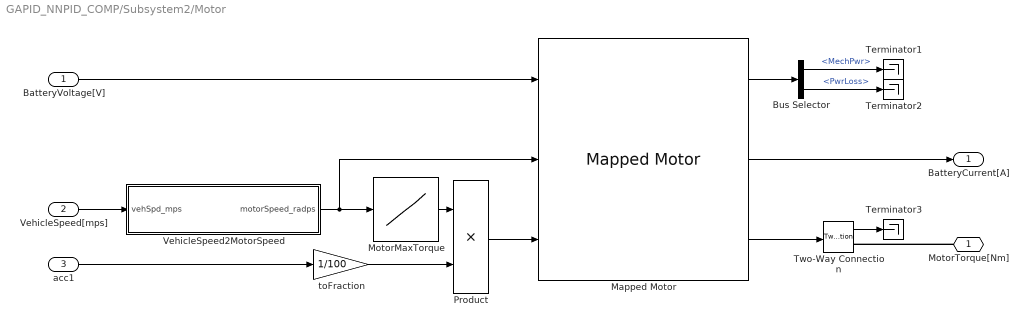
== system GAPID_NNPID_COMP/Subsystem2/Motor ==
  BatteryVoltage[V] : Inport
  VehicleSpeed[mps] : Inport  Port=2
  acc1 : Inport  Port=3
  Bus Selector : BusSelector  OutputSignals=MechPwr,PwrLoss
  Mapped Motor : autolibmappedmotor/Mapped Motor  port_config=Speed  param_by=Tabulated torque-speed envelope  w_t=motorSpeedRadPs  T_t=motorMaxTorqueNm  torque_max=.1  power_max=30  Tc=0.02  param_loss=Single efficiency measurement  eff=100  w_eff=375  T_eff=0.08  Piron=0  Pbase=0  w_eff_bp=[-8000 -4000 0 4000 8000]  T_eff_bp=[0 0.03 0.06 0.09]  losses_table=[1.49 1.67 2.21 3.10; 0.42 0.69 1.14 2.03; 0.06 0.24 0.78 1.68; 0.42 0.69 1.14 2.03; 1.49 1.67 2.21 3.10]  efficiency_table=[95 95 95 95; 95 95 95 95; 95 95 95 95; 95 95 95 95; 95 95 95 95]  J=5e-6  b=1e-5  omega_o=0  T_t_extended=[166.666666666667 178.571428571429 192.307692307692 208.333333333333 227.272727272727 250 277.777777777778 312.5 357.142857142857 416.666666666667 500 500 500 500 500 500 500 500 500 500 500 416.666666666667 357.142857142857 312.5 277.777777777778 250 227.272727272727 208.333333333333 192.307692307692 178.571428571429 166.666666666667]  w_t_extended=[-600 -560 -520 -480 -440 -400 -360 -320 -280 -240 -200 -160 -120 -80 -40 0 40 80 120 160 200 240 280 320 360 400 440 480 520 560 600]  KLossIron=0  KLossCopper=0  x_w_eff_vec=[-8000 -4000 0 4000 8000]  x_T_eff_vec=[-0.09 -0.06 -0.03 0 0.03 0.06 0.09]  x_losses_mat=[3.1 2.21 1.67 1.49 1.67 2.21 3.1;2.03 1.14 0.69 0.42 0.69 1.14 2.03;1.68 0.78 0.24 0.06 0.24 0.78 1.68;2.03 1.14 0.69 0.42 0.69 1.14 2.03;3.1 2.21 1.67 1.49 1.67 2.21 3.1]  aMode=aMode
  MotorMaxTorque : Lookup_n-D  NumberOfTableDimensions=1  BreakpointsForDimension1=motorSpeedRadPs  Table=motorMaxTorqueNm  ExtrapMethod=Clip  InternalRulePriority=Speed  RndMeth=Simplest  InputSameDT=on
  Product : Product
  Terminator1 : Terminator
  Terminator2 : Terminator
  Terminator3 : Terminator
  Two-Way Connectio n : TwoWayConnection
  VehicleSpeed2MotorSpeed : Subsystem
  toFraction : Gain  Gain=1/100
  MotorTorque[Nm] : PMIOPort  Side=Right
  BatteryCurrent[A] : Outport  VectorParamsAs1DForOutWhenUnconnected=off
  wires:
  BatteryVoltage[V]/1 -> Mapped Motor/1
  Mapped Motor/2 -> BatteryCurrent[A]/1
  VehicleSpeed[mps]/1 -> VehicleSpeed2MotorSpeed/1(vehSpd_mps)
  VehicleSpeed2MotorSpeed/1(motorSpeed_radps) -> MotorMaxTorque/1, Mapped Motor/2
  Mapped Motor/1 -> Bus Selector/1
  Two-Way Connectio n/1 -> Terminator3/1
  Product/1 -> Mapped Motor/3
  MotorMaxTorque/1 -> Product/1
  acc1/1 -> toFraction/1
  toFraction/1 -> Product/2
  Bus Selector/2 -> Terminator2/1  "<PwrLoss>"
  Bus Selector/1 -> Terminator1/1  "<MechPwr>"
  Mapped Motor/3 -> Two-Way Connectio n/1
  connections:
  MotorTorque[Nm]/RConn1 -- Two-Way Connectio n/RConn1

== system GAPID_NNPID_COMP/Subsystem2/Rear Differential ==
  Axle : autolibsharedcoupling/Torsional Compliance  port_config=Two-way connection  k=axle_k  b=axle_b  theta_o=0  domega_o=0  omega_c=bevAxle_wc  blkID=0  aMode=1
  Open Differential : autolibshareddiff/Open Differential  shaftSwitchMask=To the left of center-line  Ndiff=diffRatio  Jd=.025  bd=1e-3  Jw1=.01  bw1=1e-3  Jw2=.01  bw2=1e-3  omegaw1o=0  omegaw2o=0  maxAbsSpd=5e3  aMode=aMode
  Terminator5 : Terminator
  Terminator6 : Terminator
  Two-Way Connection1 : TwoWayConnection
  Two-Way Connection2 : TwoWayConnection
  AxleTorque[Nm] : PMIOPort  Side=Right
  TorqueInput[Nm] : PMIOPort  Port=2  Side=Left
  wires:
  Open Differential/3 -> Two-Way Connection1/1
  Open Differential/4 -> Terminator5/1
  Open Differential/1 -> Terminator6/1  "Diff"
  Open Differential/2 -> Two-Way Connection2/1
  Two-Way Connection1/1 -> Open Differential/2, Open Differential/3
  Two-Way Connection2/1 -> Open Differential/1
  connections:
  Axle/LConn1 -- Two-Way Connection1/RConn1
  TorqueInput[Nm]/RConn1 -- Two-Way Connection2/RConn1
  AxleTorque[Nm]/RConn1 -- Axle/RConn1

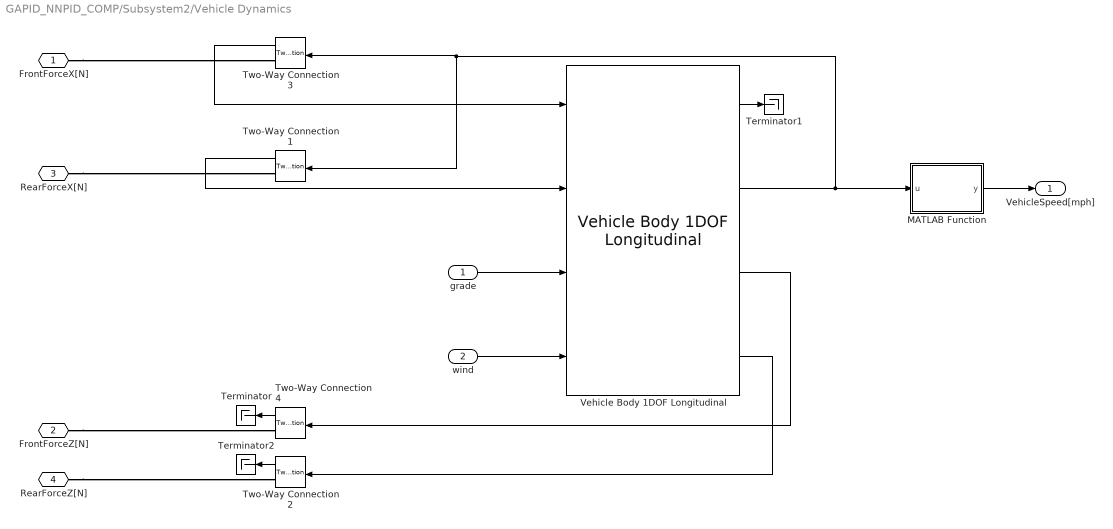
== system GAPID_NNPID_COMP/Subsystem2/Vehicle Dynamics ==
  grade : Inport
  wind : Inport  Port=2
  MATLAB Function : MATLAB Function  TreatAsAtomicUnit=on
  Terminator : Terminator
  Terminator1 : Terminator
  Terminator2 : Terminator
  Two-Way Connection{1..4} (4 alike) : TwoWayConnection
  Vehicle Body 1DOF Longitudinal : autolibshared/Vehicle Body 1DOF Longitudinal  VariantControl=SL  aMode=aMode  NF=2  NR=2  m=1468  a=1.13225  b=1.45575  h=.35  Cd=0.29  Af=2.22  x_o=0  xdot_o=0  Pabs=101325  T=293.15  g=9.81
  FrontForceX[N] : PMIOPort  Side=Left
  FrontForceZ[N] : PMIOPort  Port=2  Side=Left
  RearForceX[N] : PMIOPort  Port=3  Side=Left
  RearForceZ[N] : PMIOPort  Port=4  Side=Left
  VehicleSpeed[mph] : Outport  VectorParamsAs1DForOutWhenUnconnected=off
  wires:
  grade/1 -> Vehicle Body 1DOF Longitudinal/3
  wind/1 -> Vehicle Body 1DOF Longitudinal/4
  Vehicle Body 1DOF Longitudinal/1 -> Terminator1/1
  Vehicle Body 1DOF Longitudinal/3 -> Two-Way Connection4/1
  Vehicle Body 1DOF Longitudinal/4 -> Two-Way Connection2/1
  Two-Way Connection3/1 -> Vehicle Body 1DOF Longitudinal/1
  Two-Way Connection1/1 -> Vehicle Body 1DOF Longitudinal/2
  Two-Way Connection4/1 -> Terminator/1
  Two-Way Connection2/1 -> Terminator2/1
  Vehicle Body 1DOF Longitudinal/2 -> MATLAB Function/1(u), Two-Way Connection1/1, Two-Way Connection3/1
  MATLAB Function/1(y) -> VehicleSpeed[mph]/1
  connections:
  FrontForceX[N]/RConn1 -- Two-Way Connection3/RConn1
  FrontForceZ[N]/RConn1 -- Two-Way Connection4/RConn1
  RearForceX[N]/RConn1 -- Two-Way Connection1/RConn1
  RearForceZ[N]/RConn1 -- Two-Way Connection2/RConn1

== system GAPID_NNPID_COMP/Subsystem3/Battery ==
  LoadCurrent[A] : Inport
  AmbientTemp[C] : Constant  Value=27
  Bus Selector : BusSelector  OutputSignals=BattSoc
  C2K : Bias  Bias=273
  Datasheet Battery : autolibdatasheetbattery/Datasheet Battery  CapacityCtrl=Parameter  OutputVlt=Unfiltered  BattChargeMax=131.82  Em=[3.167 3.413 3.446 3.488 3.537 3.571 3.593 3.610 3.625 3.642 3.663 3.695 3.755 3.799 3.846 3.895 3.945 3.997 4.051 4.108 4.166]  CapLUTBp=[0 0.05 0.1 0.15 0.2 0.25 0.3 0.35 0.4 0.45 0.5 0.55 0.6 0.65 0.7 0.75 0.8 0.85 0.9 0.95 1]  RInt=[0.008846 0.009319 0.009027 0.00847 0.01032 0.01314;0.006389 0.006554 0.005553 0.005525 0.006043 0.007805;0.004364 0.004101 0.00406 0.003452 0.003846 0.004517;0.002031 0.002563 0.002532 0.00246 0.002716 0.003047;0.001443 0.001825 0.001795 0.001778 0.001924 0.002234;0.0005603 0.0007192 0.0006887 0.0007557 0.0007355 0.001014;0.001028 0.001338 0.001 0.001536 0.001546 0.002789]  BattTempBp=[243.1 253.1 263.1 273.1 283.1 298.1 313.1]  CapSOCBp=[0 0.2 0.4 0.6 0.8 1]  Ns=96  Np=2  BattCapInit=131.82  Tc=1/1000  Vinit=4.221
  SOCto% : Gain  Gain=100
  Scope : Scope
  Stop Simulation : Stop
  lowSOClimit : simulink/Logic and Bit Operations/Compare To Constant  relop=<=  const=5  OutDataTypeStr=boolean
  BatteryVoltage[V] : Outport  VectorParamsAs1DForOutWhenUnconnected=off
  wires:
  Datasheet Battery/1 -> Bus Selector/1
  AmbientTemp[C]/1 -> C2K/1
  Datasheet Battery/2 -> BatteryVoltage[V]/1
  C2K/1 -> Datasheet Battery/2
  SOCto%/1 -> lowSOClimit/1, Scope/1
  Bus Selector/1 -> SOCto%/1  "<BattSoc>"
  LoadCurrent[A]/1 -> Datasheet Battery/1
  lowSOClimit/1 -> Stop Simulation/1

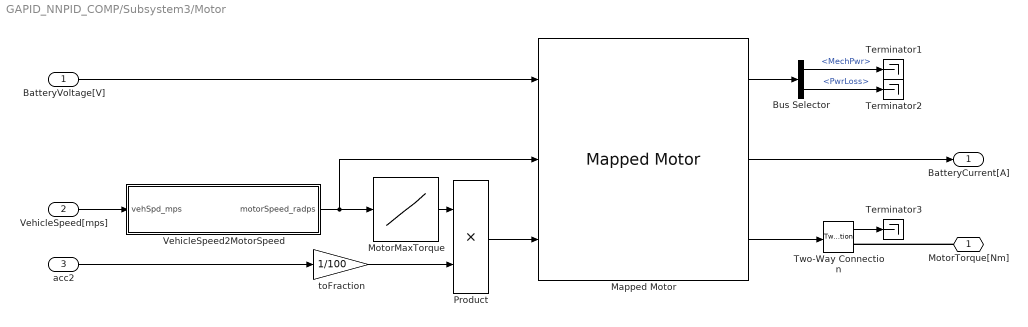
== system GAPID_NNPID_COMP/Subsystem3/Motor ==
  BatteryVoltage[V] : Inport
  VehicleSpeed[mps] : Inport  Port=2
  acc2 : Inport  Port=3
  Bus Selector : BusSelector  OutputSignals=MechPwr,PwrLoss
  Mapped Motor : autolibmappedmotor/Mapped Motor  port_config=Speed  param_by=Tabulated torque-speed envelope  w_t=motorSpeedRadPs  T_t=motorMaxTorqueNm  torque_max=.1  power_max=30  Tc=0.02  param_loss=Single efficiency measurement  eff=100  w_eff=375  T_eff=0.08  Piron=0  Pbase=0  w_eff_bp=[-8000 -4000 0 4000 8000]  T_eff_bp=[0 0.03 0.06 0.09]  losses_table=[1.49 1.67 2.21 3.10; 0.42 0.69 1.14 2.03; 0.06 0.24 0.78 1.68; 0.42 0.69 1.14 2.03; 1.49 1.67 2.21 3.10]  efficiency_table=[95 95 95 95; 95 95 95 95; 95 95 95 95; 95 95 95 95; 95 95 95 95]  J=5e-6  b=1e-5  omega_o=0  T_t_extended=[166.666666666667 178.571428571429 192.307692307692 208.333333333333 227.272727272727 250 277.777777777778 312.5 357.142857142857 416.666666666667 500 500 500 500 500 500 500 500 500 500 500 416.666666666667 357.142857142857 312.5 277.777777777778 250 227.272727272727 208.333333333333 192.307692307692 178.571428571429 166.666666666667]  w_t_extended=[-600 -560 -520 -480 -440 -400 -360 -320 -280 -240 -200 -160 -120 -80 -40 0 40 80 120 160 200 240 280 320 360 400 440 480 520 560 600]  KLossIron=0  KLossCopper=0  x_w_eff_vec=[-8000 -4000 0 4000 8000]  x_T_eff_vec=[-0.09 -0.06 -0.03 0 0.03 0.06 0.09]  x_losses_mat=[3.1 2.21 1.67 1.49 1.67 2.21 3.1;2.03 1.14 0.69 0.42 0.69 1.14 2.03;1.68 0.78 0.24 0.06 0.24 0.78 1.68;2.03 1.14 0.69 0.42 0.69 1.14 2.03;3.1 2.21 1.67 1.49 1.67 2.21 3.1]  aMode=aMode
  MotorMaxTorque : Lookup_n-D  NumberOfTableDimensions=1  BreakpointsForDimension1=motorSpeedRadPs  Table=motorMaxTorqueNm  ExtrapMethod=Clip  InternalRulePriority=Speed  RndMeth=Simplest  InputSameDT=on
  Product : Product
  Terminator1 : Terminator
  Terminator2 : Terminator
  Terminator3 : Terminator
  Two-Way Connectio n : TwoWayConnection
  VehicleSpeed2MotorSpeed : Subsystem
  toFraction : Gain  Gain=1/100
  MotorTorque[Nm] : PMIOPort  Side=Right
  BatteryCurrent[A] : Outport  VectorParamsAs1DForOutWhenUnconnected=off
  wires:
  BatteryVoltage[V]/1 -> Mapped Motor/1
  Mapped Motor/2 -> BatteryCurrent[A]/1
  VehicleSpeed[mps]/1 -> VehicleSpeed2MotorSpeed/1(vehSpd_mps)
  VehicleSpeed2MotorSpeed/1(motorSpeed_radps) -> MotorMaxTorque/1, Mapped Motor/2
  Mapped Motor/1 -> Bus Selector/1
  Two-Way Connectio n/1 -> Terminator3/1
  Product/1 -> Mapped Motor/3
  MotorMaxTorque/1 -> Product/1
  acc2/1 -> toFraction/1
  toFraction/1 -> Product/2
  Bus Selector/2 -> Terminator2/1  "<PwrLoss>"
  Bus Selector/1 -> Terminator1/1  "<MechPwr>"
  Mapped Motor/3 -> Two-Way Connectio n/1
  connections:
  MotorTorque[Nm]/RConn1 -- Two-Way Connectio n/RConn1

== system GAPID_NNPID_COMP/Subsystem3/Rear Differential ==
  Axle : autolibsharedcoupling/Torsional Compliance  port_config=Two-way connection  k=axle_k  b=axle_b  theta_o=0  domega_o=0  omega_c=bevAxle_wc  blkID=0  aMode=1
  Open Differential : autolibshareddiff/Open Differential  shaftSwitchMask=To the left of center-line  Ndiff=diffRatio  Jd=.025  bd=1e-3  Jw1=.01  bw1=1e-3  Jw2=.01  bw2=1e-3  omegaw1o=0  omegaw2o=0  maxAbsSpd=5e3  aMode=aMode
  Terminator5 : Terminator
  Terminator6 : Terminator
  Two-Way Connection1 : TwoWayConnection
  Two-Way Connection2 : TwoWayConnection
  AxleTorque[Nm] : PMIOPort  Side=Right
  TorqueInput[Nm] : PMIOPort  Port=2  Side=Left
  wires:
  Open Differential/3 -> Two-Way Connection1/1
  Open Differential/4 -> Terminator5/1
  Open Differential/1 -> Terminator6/1  "Diff"
  Open Differential/2 -> Two-Way Connection2/1
  Two-Way Connection1/1 -> Open Differential/2, Open Differential/3
  Two-Way Connection2/1 -> Open Differential/1
  connections:
  Axle/LConn1 -- Two-Way Connection1/RConn1
  TorqueInput[Nm]/RConn1 -- Two-Way Connection2/RConn1
  AxleTorque[Nm]/RConn1 -- Axle/RConn1

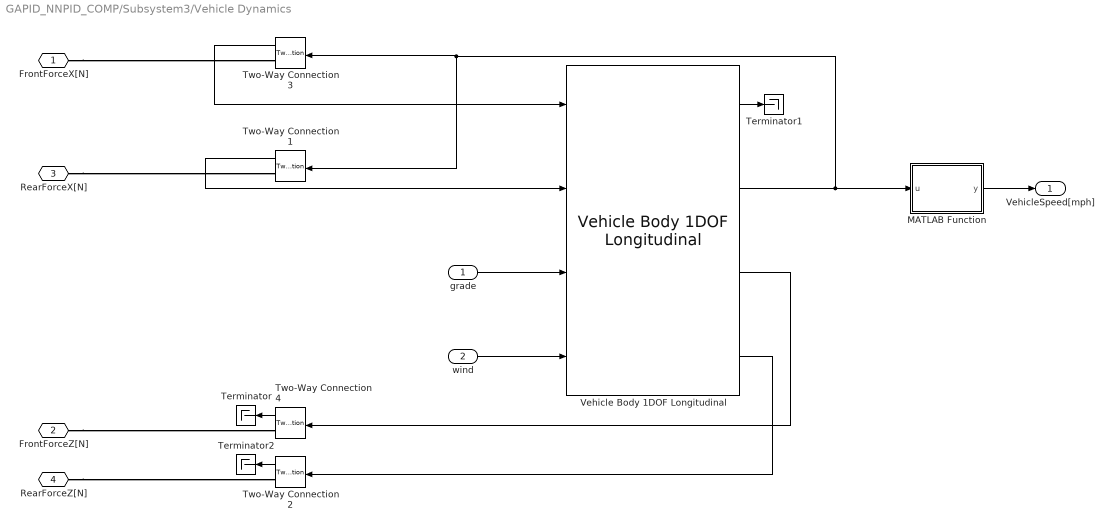
== system GAPID_NNPID_COMP/Subsystem3/Vehicle Dynamics ==
  grade : Inport
  wind : Inport  Port=2
  MATLAB Function : MATLAB Function  TreatAsAtomicUnit=on
  Terminator : Terminator
  Terminator1 : Terminator
  Terminator2 : Terminator
  Two-Way Connection{1..4} (4 alike) : TwoWayConnection
  Vehicle Body 1DOF Longitudinal : autolibshared/Vehicle Body 1DOF Longitudinal  VariantControl=SL  aMode=aMode  NF=2  NR=2  m=1468  a=1.13225  b=1.45575  h=.35  Cd=0.29  Af=2.22  x_o=0  xdot_o=0  Pabs=101325  T=293.15  g=9.81
  FrontForceX[N] : PMIOPort  Side=Left
  FrontForceZ[N] : PMIOPort  Port=2  Side=Left
  RearForceX[N] : PMIOPort  Port=3  Side=Left
  RearForceZ[N] : PMIOPort  Port=4  Side=Left
  VehicleSpeed[mph] : Outport  VectorParamsAs1DForOutWhenUnconnected=off
  wires:
  grade/1 -> Vehicle Body 1DOF Longitudinal/3
  wind/1 -> Vehicle Body 1DOF Longitudinal/4
  Vehicle Body 1DOF Longitudinal/1 -> Terminator1/1
  Vehicle Body 1DOF Longitudinal/3 -> Two-Way Connection4/1
  Vehicle Body 1DOF Longitudinal/4 -> Two-Way Connection2/1
  Two-Way Connection3/1 -> Vehicle Body 1DOF Longitudinal/1
  Two-Way Connection1/1 -> Vehicle Body 1DOF Longitudinal/2
  Two-Way Connection4/1 -> Terminator/1
  Two-Way Connection2/1 -> Terminator2/1
  Vehicle Body 1DOF Longitudinal/2 -> MATLAB Function/1(u), Two-Way Connection1/1, Two-Way Connection3/1
  MATLAB Function/1(y) -> VehicleSpeed[mph]/1
  connections:
  FrontForceX[N]/RConn1 -- Two-Way Connection3/RConn1
  FrontForceZ[N]/RConn1 -- Two-Way Connection4/RConn1
  RearForceX[N]/RConn1 -- Two-Way Connection1/RConn1
  RearForceZ[N]/RConn1 -- Two-Way Connection2/RConn1

== system GAPID_NNPID_COMP/Driver2/Subsystem/NN2 ==
  who : Inport
  wih : Inport  Port=2
  learnrate : Inport  Port=3
  u_k : Inport  Port=4
  y_k : Inport  Port=5
  ek : Inport  Port=6
  Display3 : Display
  Display4 : Display
  Unit Delay{1..4} (4 alike) : UnitDelay  SampleTime=-1  HasFrameUpgradeWarning=on
  neural network : Subsystem
  K : Outport
  wires:
  y_k/1 -> Unit Delay2/1, neural network/6(y_k)
  Unit Delay4/1 -> neural network/10(e_k2)
  Unit Delay3/1 -> neural network/5(u_k1)
  u_k/1 -> Unit Delay3/1, neural network/4(u_k)
  neural network/1(weights_input_hidden) -> Display3/1
  Unit Delay1/1 -> neural network/9(e_k1), Unit Delay4/1
  neural network/2(weights_hidden_output) -> Display4/1
  ek/1 -> neural network/8(e_k), Unit Delay1/1
  Unit Delay2/1 -> neural network/7(y_k1)
  neural network/3(K) -> K/1
  wih/1 -> neural network/2(wih)
  who/1 -> neural network/1(who)
  learnrate/1 -> neural network/3(learnrate)

== system GAPID_NNPID_COMP/Subsystem2/Motor/VehicleSpeed2MotorSpeed ==
  vehSpd_mps : Inport
  Gain1 : Gain  Gain=diffRatio
  Gain2 : Gain  Gain=1/wheelRadius
  Signal Specification1 : SignalSpecification  Unit=rad/s
  motorSpeed_radps : Outport  VectorParamsAs1DForOutWhenUnconnected=off
  wires:
  Signal Specification1/1 -> motorSpeed_radps/1
  vehSpd_mps/1 -> Gain1/1
  Gain1/1 -> Gain2/1
  Gain2/1 -> Signal Specification1/1

== system GAPID_NNPID_COMP/Subsystem3/Motor/VehicleSpeed2MotorSpeed ==
  vehSpd_mps : Inport
  Gain1 : Gain  Gain=diffRatio
  Gain2 : Gain  Gain=1/wheelRadius
  Signal Specification1 : SignalSpecification  Unit=rad/s
  motorSpeed_radps : Outport  VectorParamsAs1DForOutWhenUnconnected=off
  wires:
  Signal Specification1/1 -> motorSpeed_radps/1
  vehSpd_mps/1 -> Gain1/1
  Gain1/1 -> Gain2/1
  Gain2/1 -> Signal Specification1/1

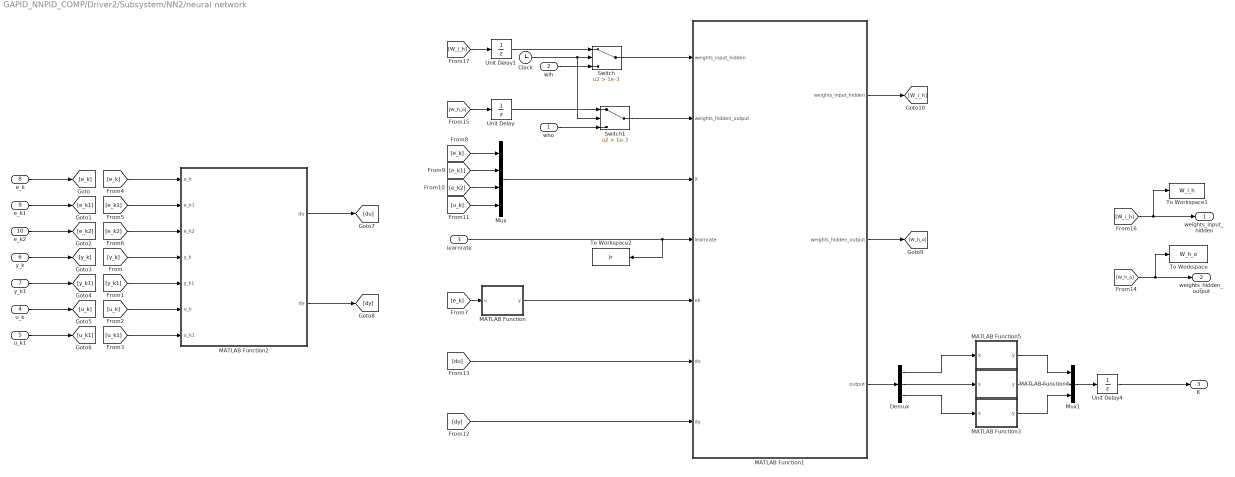
== system GAPID_NNPID_COMP/Driver2/Subsystem/NN2/neural network ==
  who : Inport
  wih : Inport  Port=2
  learnrate : Inport  Port=3
  u_k : Inport  Port=4
  u_k1 : Inport  Port=5
  y_k : Inport  Port=6
  y_k1 : Inport  Port=7
  e_k : Inport  Port=8
  e_k1 : Inport  Port=9
  e_k2 : Inport  Port=10
  Clock : Clock
  Demux : Demux  Outputs=3
  MATLAB Function : MATLAB Function  TreatAsAtomicUnit=on
  MATLAB Function1 : MATLAB Function  TreatAsAtomicUnit=on
  MATLAB Function2 : MATLAB Function  TreatAsAtomicUnit=on
  MATLAB Function3 : MATLAB Function  TreatAsAtomicUnit=on
  MATLAB Function4 : MATLAB Function  TreatAsAtomicUnit=on
  MATLAB Function5 : MATLAB Function  TreatAsAtomicUnit=on
  Mux : Mux
  Mux1 : Mux  Inputs=3
  Switch : Switch  Criteria=u2 > Threshold  Threshold=1e-3
  Switch1 : Switch  Criteria=u2 > Threshold  Threshold=1e-3
  To Workspace : ToWorkspace  VariableName=W_h_o  SampleTime=-1
      settings: MaxDataPoints=4  Save2DSignal=2-D array (concatenate along first dimension)
  To Workspace1 : ToWorkspace  VariableName=W_i_h  SampleTime=-1
      settings: MaxDataPoints=4  Save2DSignal=2-D array (concatenate along first dimension)
  To Workspace2 : ToWorkspace  VariableName=lr  SampleTime=-1
      settings: MaxDataPoints=4  Save2DSignal=2-D array (concatenate along first dimension)
  Unit Delay : UnitDelay  SampleTime=-1  HasFrameUpgradeWarning=on
  Unit Delay1 : UnitDelay  SampleTime=-1  HasFrameUpgradeWarning=on
  Unit Delay4 : UnitDelay  SampleTime=-1  HasFrameUpgradeWarning=on
  weights_input_hidden : Outport
  weights_hidden_output : Outport  Port=2
  K : Outport  Port=3
  wires:
  Switch1/1 -> MATLAB Function1/2("weights_hidden_output ")
  Mux/1 -> MATLAB Function1/3(X)
  Unit Delay/1 -> Switch1/1
  wih/1 -> Switch/3
  [e_k1] -> MATLAB Function2/2(e_k1)
  [e_k2] -> MATLAB Function2/3(e_k2)
  learnrate/1 -> MATLAB Function1/4(learnrate), To Workspace2/1
  Switch/1 -> MATLAB Function1/1("weights_input_hidden ")
  who/1 -> Switch1/3
  [y_k] -> MATLAB Function2/4(y_k)
  Clock/1 -> Switch/2, Switch1/2
  Unit Delay1/1 -> Switch/1
  [y_k1] -> MATLAB Function2/5(y_k1)
  [u_k1] -> MATLAB Function2/7(u_k1)
  Demux/1 -> MATLAB Function5/1(x)
  Demux/2 -> MATLAB Function4/1(x)
  Demux/3 -> MATLAB Function3/1(x)
  [W_h_o] -> To Workspace/1, weights_hidden_output/1
  [dy] -> MATLAB Function1/7(dy)
  MATLAB Function/1(y) -> MATLAB Function1/5(ek)
  MATLAB Function3/1(y) -> Mux1/3
  MATLAB Function4/1(y) -> Mux1/2
  MATLAB Function5/1(y) -> Mux1/1
  [u_k] -> MATLAB Function2/6(u_k)
  [du] -> MATLAB Function1/6(du)
  [e_k] -> MATLAB Function2/1(e_k)
  MATLAB Function1/3(output) -> Demux/1
  Mux1/1 -> Unit Delay4/1
  Unit Delay4/1 -> K/1
  e_k/1 -> [e_k]
  e_k1/1 -> [e_k1]
  e_k2/1 -> [e_k2]
  y_k/1 -> [y_k]
  y_k1/1 -> [y_k1]
  u_k/1 -> [u_k]
  u_k1/1 -> [u_k1]
  [e_k] -> MATLAB Function/1(u)
  [e_k] -> Mux/1
  [e_k1] -> Mux/2
  [e_k2] -> Mux/3
  [u_k] -> Mux/4
  MATLAB Function2/1(du) -> [du]
  MATLAB Function2/2(dy) -> [dy]
  MATLAB Function1/2(weights_hidden_output) -> [W_h_o]
  [W_h_o] -> Unit Delay/1
  MATLAB Function1/1(weights_input_hidden) -> [W_i_h]
  [W_i_h] -> To Workspace1/1, weights_input_hidden/1
  [W_i_h] -> Unit Delay1/1

== matlab function GAPID_NNPID_COMP/Subsystem3/Vehicle Dynamics/MATLAB Function ==
  data: u input; y output
function y = fcn(u)
if u > 10^5;
    u = 10^5;
elseif u < -10^5;
    u=-10^5;
end
y = u;

== matlab function GAPID_NNPID_COMP/Driver2/Subsystem/NN2/neural network/MATLAB Function ==
  data: u input; y output
function y = fcn(u)

y = 0.5*u^2;

== matlab function GAPID_NNPID_COMP/Driver1/MATLAB Function2 ==
  data: vw1 input; vw output double; th output fixdt('double', 'DataTypeOverride', 'Off'); th1 input; ref1 input; ref output double; a input; b input; c input
%%%%%%%%%%%%%%%%%%%%%%%%%%%%%%%%%%%%%%%%%%%%%%%%%%%%%%%%%%%%%%%%%%%%%%%%%%%
% Author: Yassine Kebbati
% Date: 20/12/2019
% Control NN_PID-GA_PID-COMPARISON
%%%%%%%%%%%%%%%%%%%%%%%%%%%%%%%%%%%%%%%%%%%%%%%%%%%%%%%%%%%%%%%%%%%%%%%%%%%
%minimum euclidean distance
function [vw,th,ref] = fcn(vw1,th1,ref1,a,b,c)
% coder.extrinsic('xlsread');
% %data = xlsread('rand_d.xls');


% th1 = reshape(data(:,4),numel(data(:,4)),1);%data(:,4);
% vw1 = reshape(data(:,5),numel(data(:,5)),1);
% ref1 = reshape(data(:,6),numel(data(:,6)),1);

% th1 = 5.21365;
% vw1 = 2.0549;
% ref1 = 1.0265;


d1 = abs(vw1-a); %sqrt((vw1-vw).^2);
d2 = abs(th1-b); %sqrt((th1-th).^2);
d3 = abs(ref1-c); %sqrt((ref1-ref).^2);

v1 = vw1(find(d1 == min(d1(:))));
v2 = th1(find(d2 == min(d2(:))));  %smallest distance
v3 = ref1(find(d3 == min(d3(:))));


vw= v1(1,1);
th= v2(1,1);
ref= v3(1,1);

== matlab function GAPID_NNPID_COMP/Driver2/Subsystem/NN2/neural network/MATLAB Function1 ==
  data: weights_input_hidden output; weights_input_hidden input; weights_hidden_output input; X input; learnrate input; ek input; weights_hidden_output output; du input; dy input; output output size=[3,1]
%%%%%%%%%%%%%%%%%%%%%%%%%%%%%%%%%%%%%%%%%%%%%%%%%%%%%%%%%%%%%%%%%%%%%%%%%%%
% Author: Yassine Kebbati
% Date: 20/12/2019
% Control NN-PID-Autonomous_Driving
%%%%%%%%%%%%%%%%%%%%%%%%%%%%%%%%%%%%%%%%%%%%%%%%%%%%%%%%%%%%%%%%%%%%%%%%%%%

function [weights_input_hidden, weights_hidden_output,output]=gradient(weights_input_hidden,weights_hidden_output,X, learnrate, ek, du,dy)


hidden_layer_in = weights_input_hidden'*X;
hidden_layer_out = sig(hidden_layer_in);



output_layer_in = weights_hidden_output'*hidden_layer_out;

output = output_layer_in;


output_error_term = ek * dy *du;


hidden_error_term = (weights_hidden_output * output_error_term) .* (hidden_layer_out.*(1 - hidden_layer_out));



delta_w_h_o = -learnrate * hidden_layer_out * output_error_term.';

delta_w_i_h = -learnrate * X * hidden_error_term.';


weights_input_hidden =  weights_input_hidden + delta_w_i_h;  

weights_hidden_output =  weights_hidden_output + delta_w_h_o;

== matlab function GAPID_NNPID_COMP/Driver2/Subsystem/NN2/neural network/MATLAB Function2 ==
  data: e_k input; du output; e_k1 input; e_k2 input; y_k input; y_k1 input; u_k input; u_k1 input; dy output
%%%%%%%%%%%%%%%%%%%%%%%%%%%%%%%%%%%%%%%%%%%%%%%%%%%%%%%%%%%%%%%%%%%%%%%%%%%
% Author: Yassine Kebbati
% Date: 20/12/2019
% Control NN-PID-Autonomous_Driving
%%%%%%%%%%%%%%%%%%%%%%%%%%%%%%%%%%%%%%%%%%%%%%%%%%%%%%%%%%%%%%%%%%%%%%%%%%%

function [du, dy] = error(e_k, e_k1, e_k2, y_k, y_k1, u_k, u_k1)
T = (1e-3);
du = [(e_k - e_k1); T/2*(e_k- e_k1) ;(e_k - 2*e_k1 + e_k2)/T]; 
%du = [(e_k - e_k1); (e_k - e_k1) ;(e_k - 2*e_k1 + e_k2)];

if (u_k - u_k1)==0
   dy = sign(y_k - y_k1); 
else
    dy = sign((y_k - y_k1)/(u_k - u_k1));
end

== matlab function GAPID_NNPID_COMP/Driver2/Subsystem/NN2/neural network/MATLAB Function3 ==
  data: x input; y output
function y = relu(x)

if x>0
    y=x;
else
    y=0;
end

== matlab function GAPID_NNPID_COMP/Driver2/Subsystem/NN2/neural network/MATLAB Function4 ==
  data: x input; y output
function y = relu(x)

if x>0
    y=x;
else
    y=0;
end

== matlab function GAPID_NNPID_COMP/Driver2/Subsystem/NN2/neural network/MATLAB Function5 ==
  data: x input; y output

function y = relu(x)

if x>0
    y=x;
else
    y=0;
end

== matlab function GAPID_NNPID_COMP/Subsystem2/Vehicle Dynamics/MATLAB Function ==
  data: u input; y output
function y = fcn(u)
if u > 10^5;
    u = 10^5;
elseif u < -10^5;
    u=-10^5;
end
y = u;
